simulink model "demo2"  (R2022a)
settings: Solver=ode45  StartTime=0.0  StopTime=inf  RelTol=1e-3  EnableMultiTasking=on
values from neighbouring files (symbols this model uses):
  Cf = 435.418/0.296296    (= 1469.53721954)    [demo2_CM.m]
  controlConstraints = [ ... (first row only)    [demo2_CM.m]
  controlWeight = [1e-7 1e-10 1e-10]    [demo2_CM.m]
  Cr = 756.349/(0.6*pi/180)    (= 72226.0092316)    [demo2_CM.m]
  initial_input = [0 0 0]'    [demo2_CM.m]
  initial_state = [50/3.6 0 0]'    [demo2_CM.m]
  Iz = 2488.892    [demo2_CM.m]
  Kd = 0.0    (= 0)    [demo2_CM.m]
  Ki = 5    [demo2_CM.m]
  Kp = 0.000000005    (= 5e-09)    [demo2_CM.m]
  lf = 1.240    (= 1.24)    [demo2_CM.m]
  lr = 1.510    (= 1.51)    [demo2_CM.m]
  m = 1644.80    (= 1644.8)    [demo2_CM.m]
  Nc = 1    [demo2_CM.m]
  Np = 20    [demo2_CM.m]
  stateConstraints = [ ... (first row only)    [demo2_CM.m]
  stateWeight = [1 1 5]    [demo2_CM.m]
  Ts = 0.01    [demo2_CM.m]
  Vx_ref = 60 / 3.6    (= 16.6666666667)    [demo2_CM.m]
  Vy_ref = 0    [demo2_CM.m]
  w = 0.8    [demo2_CM.m]
  YawRate_ref = -0.006    [demo2_CM.m]
undefined symbols (not defined in the file or in its folder): DiscIntNeverNeededParam, steer
libraries: CarMaker4SL x14, slpidlib x2, simulink x1
(part 2 of 2)

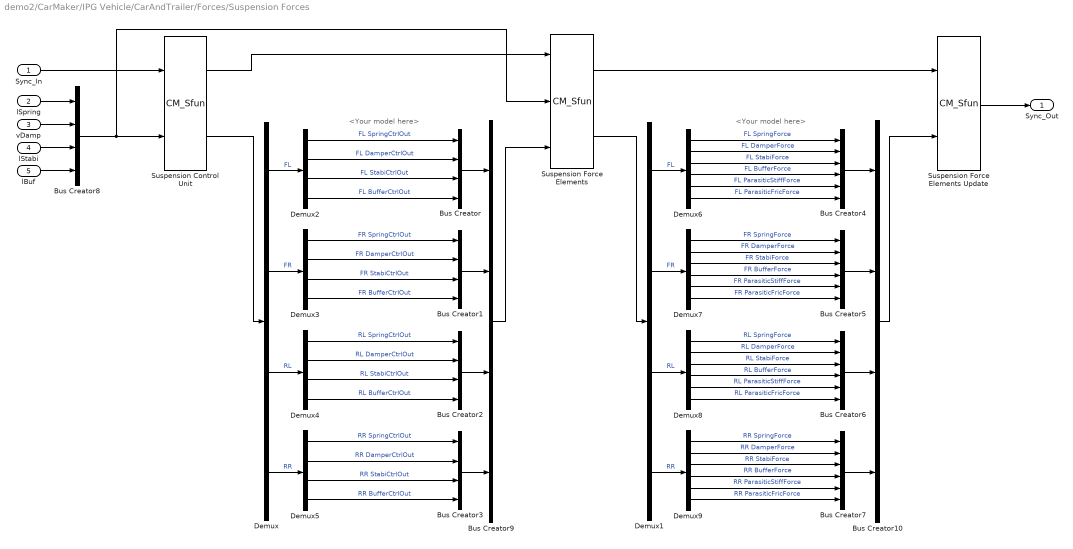
== system demo2/CarMaker/IPG Vehicle/CarAndTrailer/Forces/Suspension Forces ==
  note: <Your model here>
  note: <Your model here>
  Sync_In : Inport
  lSpring : Inport  Port=2
  vDamp : Inport  Port=3
  lStabi : Inport  Port=4
  lBuf : Inport  Port=5
  Bus Creator{,1..3,8..10} (7 alike) : BusCreator  Inputs=4
  Bus Creator{4..7} (4 alike) : BusCreator  Inputs=6
  Demux{,1..5} (6 alike) : Demux
  Demux{6..9} (4 alike) : Demux  Outputs=6
  Suspension Control Unit : S-Function  FunctionName=CM_Sfun  Parameters='ForcesSuspControl'  SFunctionDeploymentMode=off  EnableBusSupport=off
  Suspension Force Elements : S-Function  FunctionName=CM_Sfun  Parameters='ForcesSusp'  SFunctionDeploymentMode=off  EnableBusSupport=off
  Suspension Force Elements Update : S-Function  FunctionName=CM_Sfun  Parameters='ForcesSuspUpd'  SFunctionDeploymentMode=off  EnableBusSupport=off
  Sync_Out : Outport  VectorParamsAs1DForOutWhenUnconnected=off
  wires:
  vDamp/1 -> Bus Creator8/2
  lStabi/1 -> Bus Creator8/3
  lBuf/1 -> Bus Creator8/4
  lSpring/1 -> Bus Creator8/1
  Bus Creator8/1 -> Suspension Control Unit/2, Suspension Force Elements/2
  Sync_In/1 -> Suspension Control Unit/1
  Suspension Control Unit/1 -> Suspension Force Elements/1
  Suspension Force Elements/1 -> Suspension Force Elements Update/1
  Suspension Force Elements Update/1 -> Sync_Out/1
  Bus Creator4/1 -> Bus Creator10/1
  Bus Creator5/1 -> Bus Creator10/2
  Bus Creator6/1 -> Bus Creator10/3
  Bus Creator7/1 -> Bus Creator10/4
  Demux6/1 -> Bus Creator4/1  "FL SpringForce"
  Demux9/1 -> Bus Creator7/1  "RR SpringForce"
  Demux9/2 -> Bus Creator7/2  "RR DamperForce"
  Demux9/3 -> Bus Creator7/3  "RR StabiForce"
  Demux9/4 -> Bus Creator7/4  "RR BufferForce"
  Demux9/5 -> Bus Creator7/5  "RR ParasiticStiffForce"
  Demux9/6 -> Bus Creator7/6  "RR ParasiticFricForce"
  Demux8/1 -> Bus Creator6/1  "RL SpringForce"
  Demux8/2 -> Bus Creator6/2  "RL DamperForce"
  Demux8/4 -> Bus Creator6/4  "RL BufferForce"
  Demux8/5 -> Bus Creator6/5  "RL ParasiticStiffForce"
  Demux8/6 -> Bus Creator6/6  "RL ParasiticFricForce"
  Demux8/3 -> Bus Creator6/3  "RL StabiForce"
  Demux7/1 -> Bus Creator5/1  "FR SpringForce"
  Demux7/2 -> Bus Creator5/2  "FR DamperForce"
  Demux7/3 -> Bus Creator5/3  "FR StabiForce"
  Demux7/4 -> Bus Creator5/4  "FR BufferForce"
  Demux7/5 -> Bus Creator5/5  "FR ParasiticStiffForce"
  Demux7/6 -> Bus Creator5/6  "FR ParasiticFricForce"
  Demux6/2 -> Bus Creator4/2  "FL DamperForce"
  Demux6/3 -> Bus Creator4/3  "FL StabiForce"
  Demux6/4 -> Bus Creator4/4  "FL BufferForce"
  Demux6/5 -> Bus Creator4/5  "FL ParasiticStiffForce"
  Demux6/6 -> Bus Creator4/6  "FL ParasiticFricForce"
  Bus Creator10/1 -> Suspension Force Elements Update/2
  Demux/1 -> Demux2/1  "FL"
  Bus Creator1/1 -> Bus Creator9/2
  Demux/2 -> Demux3/1  "FR"
  Bus Creator2/1 -> Bus Creator9/3
  Demux/3 -> Demux4/1  "RL"
  Bus Creator3/1 -> Bus Creator9/4
  Demux2/1 -> Bus Creator/1  "FL SpringCtrlOut"
  Demux/4 -> Demux5/1  "RR"
  Demux5/1 -> Bus Creator3/1  "RR SpringCtrlOut"
  Demux5/2 -> Bus Creator3/2  "RR DamperCtrlOut"
  Demux5/3 -> Bus Creator3/3  "RR StabiCtrlOut"
  Demux5/4 -> Bus Creator3/4  "RR BufferCtrlOut"
  Demux4/1 -> Bus Creator2/1  "RL SpringCtrlOut"
  Demux4/2 -> Bus Creator2/2  "RL DamperCtrlOut"
  Demux4/4 -> Bus Creator2/4  "RL BufferCtrlOut"
  Demux4/3 -> Bus Creator2/3  "RL StabiCtrlOut"
  Demux3/1 -> Bus Creator1/1  "FR SpringCtrlOut"
  Demux3/2 -> Bus Creator1/2  "FR DamperCtrlOut"
  Demux3/3 -> Bus Creator1/3  "FR StabiCtrlOut"
  Demux3/4 -> Bus Creator1/4  "FR BufferCtrlOut"
  Demux2/2 -> Bus Creator/2  "FL DamperCtrlOut"
  Demux2/3 -> Bus Creator/3  "FL StabiCtrlOut"
  Demux2/4 -> Bus Creator/4  "FL BufferCtrlOut"
  Suspension Control Unit/2 -> Demux/1
  Bus Creator9/1 -> Suspension Force Elements/3
  Bus Creator/1 -> Bus Creator9/1
  Suspension Force Elements/2 -> Demux1/1
  Demux1/1 -> Demux6/1  "FL"
  Demux1/2 -> Demux7/1  "FR"
  Demux1/3 -> Demux8/1  "RL"
  Demux1/4 -> Demux9/1  "RR"

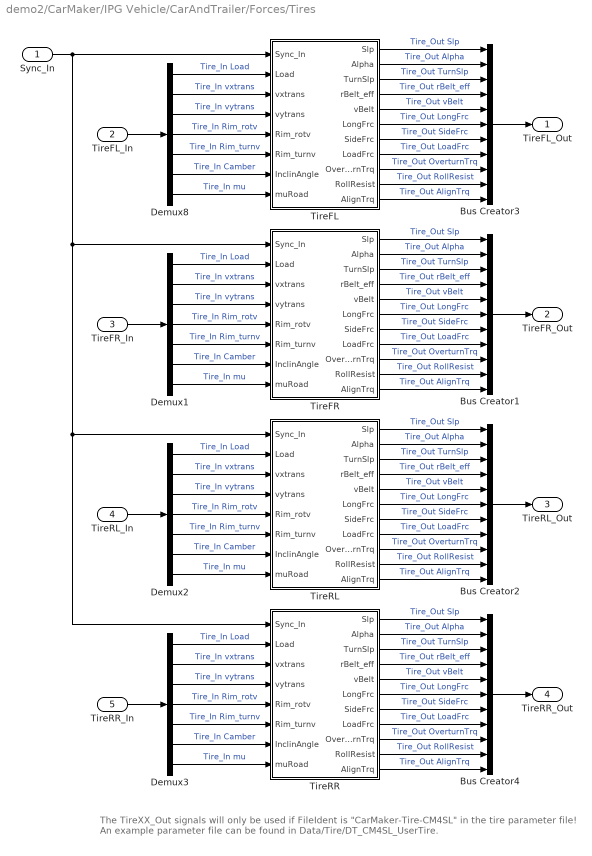
== system demo2/CarMaker/IPG Vehicle/CarAndTrailer/Forces/Tires ==
  note: The TireXX_Out signals will only be used if FileIdent is "CarMaker-Tire-CM4SL" in the tire parameter file!
      | An example parameter file can be found in Data/Tire/DT_CM4SL_UserTire.
  Sync_In : Inport
  TireFL_In : Inport  Port=2
  TireFR_In : Inport  Port=3
  TireRL_In : Inport  Port=4
  TireRR_In : Inport  Port=5
  Bus Creator{1..4} (4 alike) : BusCreator  Inputs=11
  Demux{1..3,8} (4 alike) : Demux  Outputs=7
      settings: DisplayOption=none
  TireFL : Subsystem
  TireFR : Subsystem
  TireRL : Subsystem
  TireRR : Subsystem
  TireFL_Out : Outport  VectorParamsAs1DForOutWhenUnconnected=off
  TireFR_Out : Outport  Port=2  VectorParamsAs1DForOutWhenUnconnected=off
  TireRL_Out : Outport  Port=3  VectorParamsAs1DForOutWhenUnconnected=off
  TireRR_Out : Outport  Port=4  VectorParamsAs1DForOutWhenUnconnected=off
  wires:
  Sync_In/1 -> TireRR/1(Sync_In), TireRL/1(Sync_In), TireFR/1(Sync_In), TireFL/1(Sync_In)
  Bus Creator4/1 -> TireRR_Out/1
  Bus Creator2/1 -> TireRL_Out/1
  Bus Creator1/1 -> TireFR_Out/1
  Demux3/5 -> TireRR/6(Rim_turnv)  "Tire_In Rim_turnv"
  Demux3/4 -> TireRR/5(Rim_rotv)  "Tire_In Rim_rotv"
  Demux3/1 -> TireRR/2(Load)  "Tire_In Load"
  Demux3/7 -> TireRR/8(muRoad)  "Tire_In mu"
  Demux3/6 -> TireRR/7(InclinAngle)  "Tire_In Camber"
  Demux3/2 -> TireRR/3(vxtrans)  "Tire_In vxtrans"
  Demux3/3 -> TireRR/4(vytrans)  "Tire_In vytrans"
  TireRR/11(AlignTrq) -> Bus Creator4/11  "Tire_Out AlignTrq"
  TireRR/10(RollResist) -> Bus Creator4/10  "Tire_Out RollResist"
  TireRR/9(OverturnTrq) -> Bus Creator4/9  "Tire_Out OverturnTrq"
  TireRR/8(LoadFrc) -> Bus Creator4/8  "Tire_Out LoadFrc"
  TireRR/7(SideFrc) -> Bus Creator4/7  "Tire_Out SideFrc"
  TireRR/6(LongFrc) -> Bus Creator4/6  "Tire_Out LongFrc"
  TireRR/5(vBelt) -> Bus Creator4/5  "Tire_Out vBelt"
  TireRR/4(rBelt_eff) -> Bus Creator4/4  "Tire_Out rBelt_eff"
  TireRR/3(TurnSlp) -> Bus Creator4/3  "Tire_Out TurnSlp"
  TireRR/1(Slp) -> Bus Creator4/1  "Tire_Out Slp"
  TireRR/2(Alpha) -> Bus Creator4/2  "Tire_Out Alpha"
  Demux2/5 -> TireRL/6(Rim_turnv)  "Tire_In Rim_turnv"
  Demux2/4 -> TireRL/5(Rim_rotv)  "Tire_In Rim_rotv"
  Demux2/1 -> TireRL/2(Load)  "Tire_In Load"
  Demux2/7 -> TireRL/8(muRoad)  "Tire_In mu"
  Demux2/6 -> TireRL/7(InclinAngle)  "Tire_In Camber"
  Demux2/2 -> TireRL/3(vxtrans)  "Tire_In vxtrans"
  Demux2/3 -> TireRL/4(vytrans)  "Tire_In vytrans"
  TireRL/11(AlignTrq) -> Bus Creator2/11  "Tire_Out AlignTrq"
  TireRL/10(RollResist) -> Bus Creator2/10  "Tire_Out RollResist"
  TireRL/9(OverturnTrq) -> Bus Creator2/9  "Tire_Out OverturnTrq"
  TireRL/8(LoadFrc) -> Bus Creator2/8  "Tire_Out LoadFrc"
  TireRL/7(SideFrc) -> Bus Creator2/7  "Tire_Out SideFrc"
  TireRL/6(LongFrc) -> Bus Creator2/6  "Tire_Out LongFrc"
  TireRL/5(vBelt) -> Bus Creator2/5  "Tire_Out vBelt"
  TireRL/4(rBelt_eff) -> Bus Creator2/4  "Tire_Out rBelt_eff"
  TireRL/3(TurnSlp) -> Bus Creator2/3  "Tire_Out TurnSlp"
  TireRL/1(Slp) -> Bus Creator2/1  "Tire_Out Slp"
  TireRL/2(Alpha) -> Bus Creator2/2  "Tire_Out Alpha"
  Demux1/5 -> TireFR/6(Rim_turnv)  "Tire_In Rim_turnv"
  Demux1/4 -> TireFR/5(Rim_rotv)  "Tire_In Rim_rotv"
  Demux1/1 -> TireFR/2(Load)  "Tire_In Load"
  Demux1/7 -> TireFR/8(muRoad)  "Tire_In mu"
  Demux1/6 -> TireFR/7(InclinAngle)  "Tire_In Camber"
  Demux1/2 -> TireFR/3(vxtrans)  "Tire_In vxtrans"
  Demux1/3 -> TireFR/4(vytrans)  "Tire_In vytrans"
  TireFR/11(AlignTrq) -> Bus Creator1/11  "Tire_Out AlignTrq"
  TireFR/10(RollResist) -> Bus Creator1/10  "Tire_Out RollResist"
  TireFR/9(OverturnTrq) -> Bus Creator1/9  "Tire_Out OverturnTrq"
  TireFR/8(LoadFrc) -> Bus Creator1/8  "Tire_Out LoadFrc"
  TireFR/7(SideFrc) -> Bus Creator1/7  "Tire_Out SideFrc"
  TireFR/6(LongFrc) -> Bus Creator1/6  "Tire_Out LongFrc"
  TireFR/5(vBelt) -> Bus Creator1/5  "Tire_Out vBelt"
  TireFR/4(rBelt_eff) -> Bus Creator1/4  "Tire_Out rBelt_eff"
  TireFR/3(TurnSlp) -> Bus Creator1/3  "Tire_Out TurnSlp"
  TireFR/1(Slp) -> Bus Creator1/1  "Tire_Out Slp"
  TireFR/2(Alpha) -> Bus Creator1/2  "Tire_Out Alpha"
  Demux8/5 -> TireFL/6(Rim_turnv)  "Tire_In Rim_turnv"
  Demux8/4 -> TireFL/5(Rim_rotv)  "Tire_In Rim_rotv"
  TireFL_In/1 -> Demux8/1
  Demux8/1 -> TireFL/2(Load)  "Tire_In Load"
  Demux8/7 -> TireFL/8(muRoad)  "Tire_In mu"
  Demux8/6 -> TireFL/7(InclinAngle)  "Tire_In Camber"
  Demux8/2 -> TireFL/3(vxtrans)  "Tire_In vxtrans"
  Demux8/3 -> TireFL/4(vytrans)  "Tire_In vytrans"
  TireFL/11(AlignTrq) -> Bus Creator3/11  "Tire_Out AlignTrq"
  TireFL/10(RollResist) -> Bus Creator3/10  "Tire_Out RollResist"
  TireFL/9(OverturnTrq) -> Bus Creator3/9  "Tire_Out OverturnTrq"
  TireFL/8(LoadFrc) -> Bus Creator3/8  "Tire_Out LoadFrc"
  TireFL/7(SideFrc) -> Bus Creator3/7  "Tire_Out SideFrc"
  TireFL/6(LongFrc) -> Bus Creator3/6  "Tire_Out LongFrc"
  TireFL/5(vBelt) -> Bus Creator3/5  "Tire_Out vBelt"
  TireFL/4(rBelt_eff) -> Bus Creator3/4  "Tire_Out rBelt_eff"
  TireFL/3(TurnSlp) -> Bus Creator3/3  "Tire_Out TurnSlp"
  TireFL/1(Slp) -> Bus Creator3/1  "Tire_Out Slp"
  TireFL/2(Alpha) -> Bus Creator3/2  "Tire_Out Alpha"
  Bus Creator3/1 -> TireFL_Out/1
  TireFR_In/1 -> Demux1/1
  TireRL_In/1 -> Demux2/1
  TireRR_In/1 -> Demux3/1

== system demo2/CarMaker/IPG Vehicle/CarAndTrailer/Forces/Vehicle Forces ==
  Sync_In : Inport
  Bus Creator1 : BusCreator  Inputs=12
  Bus Creator8 : BusCreator  Inputs=16
  BusCreator1 : BusCreator  Inputs=4
  BusCreator2 : BusCreator  Inputs=9
  Demux : Demux  Outputs=16
      settings: DisplayOption=none
  Demux1 : Demux  Outputs=12
      settings: DisplayOption=none
  Demux2 : Demux  Outputs=13
      settings: DisplayOption=none
  Forces : S-Function  FunctionName=CM_Sfun  Parameters='Forces'  SFunctionDeploymentMode=off  EnableBusSupport=off
  Terminator : Terminator
  Sync_Out : Outport  VectorParamsAs1DForOutWhenUnconnected=off
  Car.Virtual : Outport  Port=2  VectorParamsAs1DForOutWhenUnconnected=off
  Car.Aero : Outport  Port=3  VectorParamsAs1DForOutWhenUnconnected=off
  Car.Load : Outport  Port=4  VectorParamsAs1DForOutWhenUnconnected=off
  wires:
  BusCreator1/1 -> Terminator/1  "Aero IF (in)"
  Demux2/13 -> BusCreator2/9  "car Aero Trq_1 z"
  Demux2/12 -> BusCreator2/8  "car Aero Trq_1 y"
  Demux2/11 -> BusCreator2/7  "car Aero Trq_1 x"
  Demux2/10 -> BusCreator2/6  "car Aero Frc_1 z"
  Demux2/9 -> BusCreator2/5  "car Aero Frc_1 y"
  Demux2/8 -> BusCreator2/4  "car Aero Frc_1 x"
  Demux2/7 -> BusCreator2/3  "car Aero PoA_1 z"
  Demux2/6 -> BusCreator2/2  "car Aero PoA_1 y"
  Demux2/5 -> BusCreator2/1  "car Aero PoA_1 x"
  Demux2/4 -> BusCreator1/4  "car Aero tau_1"
  Demux2/3 -> BusCreator1/3  "car Aero ApproachVel_1 z"
  Demux2/2 -> BusCreator1/2  "car Aero ApproachVel_1 y"
  Demux2/1 -> BusCreator1/1  "car Aero ApproachVel_1 x"
  Demux/16 -> Bus Creator8/16  "Car Load_3 tz"
  Demux/15 -> Bus Creator8/15  "Car Load_3 ty"
  Demux/14 -> Bus Creator8/14  "Car Load_3 tx"
  Demux/13 -> Bus Creator8/13  "Car Load_3 mass"
  Demux1/12 -> Bus Creator1/12  "Car Virtual Trq_0 z"
  Demux1/11 -> Bus Creator1/11  "Car Virtual Trq_0 y"
  Demux1/10 -> Bus Creator1/10  "Car Virtual Trq_0 x"
  Demux1/9 -> Bus Creator1/9  "Car Virtual Trq_1 z"
  Demux1/8 -> Bus Creator1/8  "Car Virtual Trq_1 y"
  Demux1/7 -> Bus Creator1/7  "Car Virtual Trq_1 x"
  Demux1/6 -> Bus Creator1/6  "Car Virtual Frc_0 z"
  Demux1/5 -> Bus Creator1/5  "Car Virtual Frc_0 y"
  Demux1/4 -> Bus Creator1/4  "Car Virtual Frc_0 x"
  Sync_In/1 -> Forces/1
  Forces/1 -> Sync_Out/1
  BusCreator2/1 -> Car.Aero/1
  Demux1/1 -> Bus Creator1/1  "Car Virtual Frc_1 x"
  Demux1/2 -> Bus Creator1/2  "Car Virtual Frc_1 y"
  Demux1/3 -> Bus Creator1/3  "Car Virtual Frc_1 z"
  Forces/3 -> Demux2/1
  Forces/2 -> Demux1/1
  Bus Creator1/1 -> Car.Virtual/1
  Bus Creator8/1 -> Car.Load/1
  Demux/1 -> Bus Creator8/1  "Car Load_0 mass"
  Demux/2 -> Bus Creator8/2  "Car Load_0 tx"
  Demux/3 -> Bus Creator8/3  "Car Load_0 ty"
  Demux/4 -> Bus Creator8/4  "Car Load_0 tz"
  Demux/5 -> Bus Creator8/5  "Car Load_1 mass"
  Demux/6 -> Bus Creator8/6  "Car Load_1 tx"
  Demux/7 -> Bus Creator8/7  "Car Load_1 ty"
  Demux/8 -> Bus Creator8/8  "Car Load_1 tz"
  Demux/9 -> Bus Creator8/9  "Car Load_2 mass"
  Demux/10 -> Bus Creator8/10  "Car Load_2 tx"
  Demux/11 -> Bus Creator8/11  "Car Load_2 ty"
  Demux/12 -> Bus Creator8/12  "Car Load_2 tz"
  Forces/4 -> Demux/1

== system demo2/CarMaker/IPG Vehicle/CarAndTrailer/Trailer/CreateBus Car.Hitch.FrcTrq ==
  In1 : Inport
  Bus Creator7 : BusCreator  Inputs=6
  Demux7 : Demux  Outputs=6
      settings: DisplayOption=none
  Out1 : Outport  VectorParamsAs1DForOutWhenUnconnected=off
  wires:
  In1/1 -> Demux7/1
  Bus Creator7/1 -> Out1/1
  Demux7/6 -> Bus Creator7/6  "Car Hitch Trq2Car z"
  Demux7/5 -> Bus Creator7/5  "Car Hitch Trq2Car y"
  Demux7/4 -> Bus Creator7/4  "Car Hitch Trq2Car x"
  Demux7/3 -> Bus Creator7/3  "Car Hitch Frc2Car z"
  Demux7/2 -> Bus Creator7/2  "Car Hitch Frc2Car y"
  Demux7/1 -> Bus Creator7/1  "Car Hitch Frc2Car x"

== system demo2/CarMaker/IPG Vehicle/CarAndTrailer/Trailer/CreateBus Vhcl.Motion ==
  In1 : Inport
  BusCreator : BusCreator  Inputs=15
  Demux : Demux  Outputs=15
      settings: DisplayOption=none
  Out1 : Outport  VectorParamsAs1DForOutWhenUnconnected=off
  wires:
  Demux/15 -> BusCreator/15  "Vhcl YawAcc"
  Demux/14 -> BusCreator/14  "Vhcl YawVel"
  Demux/13 -> BusCreator/13  "Vhcl Yaw"
  Demux/12 -> BusCreator/12  "Vhcl PitchAcc"
  Demux/11 -> BusCreator/11  "Vhcl PitchVel"
  Demux/10 -> BusCreator/10  "Vhcl Pitch"
  Demux/9 -> BusCreator/9  "Vhcl RollAcc"
  Demux/8 -> BusCreator/8  "Vhcl RollVel"
  Demux/7 -> BusCreator/7  "Vhcl Roll"
  Demux/6 -> BusCreator/6  "Vhcl Hitch_Pos z"
  Demux/5 -> BusCreator/5  "Vhcl Hitch_Pos y"
  Demux/4 -> BusCreator/4  "Vhcl Hitch_Pos x"
  Demux/3 -> BusCreator/3  "Vhcl sRoad"
  Demux/2 -> BusCreator/2  "Vhcl Distance"
  Demux/1 -> BusCreator/1  "Vhcl v"
  In1/1 -> Demux/1
  BusCreator/1 -> Out1/1

== system demo2/CarMaker/IPG Vehicle/CarAndTrailer/Trailer/CreateBus Vhcl.PoI ==
  In1 : Inport
  Bus Creator3 : BusCreator  Inputs=18
  Demux3 : Demux  Outputs=18
      settings: DisplayOption=none
  Out1 : Outport  VectorParamsAs1DForOutWhenUnconnected=off
  wires:
  Demux3/18 -> Bus Creator3/18  "Vhcl PoI_GCS Elev"
  Demux3/17 -> Bus Creator3/17  "Vhcl PoI_GCS Lat"
  Demux3/16 -> Bus Creator3/16  "Vhcl PoI_GCS Long"
  Demux3/15 -> Bus Creator3/15  "Vhcl PoI_Acc_1 z"
  Demux3/14 -> Bus Creator3/14  "Vhcl PoI_Acc_1 y"
  Demux3/13 -> Bus Creator3/13  "Vhcl PoI_Acc_1 x"
  Demux3/12 -> Bus Creator3/12  "Vhcl PoI_Vel_1 z"
  Demux3/11 -> Bus Creator3/11  "Vhcl PoI_Vel_1 y"
  Demux3/10 -> Bus Creator3/10  "Vhcl PoI_Vel_1 x"
  Demux3/9 -> Bus Creator3/9  "Vhcl PoI_Acc z"
  Demux3/8 -> Bus Creator3/8  "Vhcl PoI_Acc y"
  Demux3/7 -> Bus Creator3/7  "Vhcl PoI_Acc x"
  Demux3/6 -> Bus Creator3/6  "Vhcl PoI_Vel z"
  Demux3/5 -> Bus Creator3/5  "Vhcl PoI_Vel y"
  Demux3/4 -> Bus Creator3/4  "Vhcl PoI_Vel x"
  Demux3/3 -> Bus Creator3/3  "Vhcl PoI_Pos z"
  Demux3/2 -> Bus Creator3/2  "Vhcl PoI_Pos y"
  In1/1 -> Demux3/1
  Bus Creator3/1 -> Out1/1
  Demux3/1 -> Bus Creator3/1  "Vhcl PoI_Pos x"

== system demo2/CarMaker/IPG Vehicle/CarAndTrailer/Trailer/CreateBus Vhcl.Steering ==
  In1 : Inport
  Bus Creator3 : BusCreator  Inputs=4
  Demux : Demux
      settings: DisplayOption=none
  Out1 : Outport  VectorParamsAs1DForOutWhenUnconnected=off
  wires:
  Bus Creator3/1 -> Out1/1
  Demux/1 -> Bus Creator3/1  "Vhcl Steering Ang"
  Demux/3 -> Bus Creator3/3  "Vhcl Steering AngAcc"
  Demux/2 -> Bus Creator3/2  "Vhcl Steering AngVel"
  Demux/4 -> Bus Creator3/4  "Vhcl Steering Trq"
  In1/1 -> Demux/1

== system demo2/CarMaker/IPG Vehicle/CarAndTrailer/Trailer/CreateBus Vhcl.Wheel.FL ==
  In1 : Inport
  Bus Creator3 : BusCreator  Inputs=14
  Demux3 : Demux  Outputs=14
      settings: DisplayOption=none
  Out1 : Outport  VectorParamsAs1DForOutWhenUnconnected=off
  wires:
  Demux3/14 -> Bus Creator3/14  "Vhcl Wheel FL Trq_WhlBearing"
  Demux3/13 -> Bus Creator3/13  "Vhcl Wheel FL Trq_T2W"
  Demux3/12 -> Bus Creator3/12  "Vhcl Wheel FL SideSlip"
  Demux3/11 -> Bus Creator3/11  "Vhcl Wheel FL LongSlip"
  Demux3/10 -> Bus Creator3/10  "Vhcl Wheel FL vBelt"
  Demux3/9 -> Bus Creator3/9  "Vhcl Wheel FL Fz"
  Demux3/8 -> Bus Creator3/8  "Vhcl Wheel FL Fy"
  Demux3/7 -> Bus Creator3/7  "Vhcl Wheel FL F"
  Demux3/6 -> Bus Creator3/6  "Vhcl Wheel FL r_zxy z"
  Demux3/5 -> Bus Creator3/5  "Vhcl Wheel FL r_zxy y"
  Demux3/4 -> Bus Creator3/4  "Vhcl Wheel FL r_zxy x"
  Demux3/3 -> Bus Creator3/3  "Vhcl Wheel FL t z"
  Demux3/2 -> Bus Creator3/2  "Vhcl Wheel FL t y"
  In1/1 -> Demux3/1
  Bus Creator3/1 -> Out1/1
  Demux3/1 -> Bus Creator3/1  "Vhcl Wheel FL t x"

== system demo2/CarMaker/IPG Vehicle/CarAndTrailer/Trailer/CreateBus Vhcl.Wheel.FR ==
  In1 : Inport
  Bus Creator3 : BusCreator  Inputs=14
  Demux3 : Demux  Outputs=14
      settings: DisplayOption=none
  Out1 : Outport  VectorParamsAs1DForOutWhenUnconnected=off
  wires:
  Demux3/14 -> Bus Creator3/14  "Vhcl Wheel FR Trq_WhlBearing"
  Demux3/13 -> Bus Creator3/13  "Vhcl Wheel FR Trq_T2W"
  Demux3/12 -> Bus Creator3/12  "Vhcl Wheel FR SideSlip"
  Demux3/11 -> Bus Creator3/11  "Vhcl Wheel FR LongSlip"
  Demux3/10 -> Bus Creator3/10  "Vhcl Wheel FR vBelt"
  Demux3/9 -> Bus Creator3/9  "Vhcl Wheel FR Fz"
  Demux3/8 -> Bus Creator3/8  "Vhcl Wheel FR Fy"
  Demux3/7 -> Bus Creator3/7  "Vhcl Wheel FR Fx"
  Demux3/6 -> Bus Creator3/6  "Vhcl Wheel FR r_zxy z"
  Demux3/5 -> Bus Creator3/5  "Vhcl Wheel FR r_zxy y"
  Demux3/4 -> Bus Creator3/4  "Vhcl Wheel FR r_zxy x"
  Demux3/3 -> Bus Creator3/3  "Vhcl Wheel FR t z"
  Demux3/2 -> Bus Creator3/2  "Vhcl Wheel FR t y"
  In1/1 -> Demux3/1
  Bus Creator3/1 -> Out1/1
  Demux3/1 -> Bus Creator3/1  "Vhcl Wheel FR t x"

== system demo2/CarMaker/IPG Vehicle/CarAndTrailer/Trailer/CreateBus Vhcl.Wheel.RL ==
  In1 : Inport
  Bus Creator3 : BusCreator  Inputs=14
  Demux3 : Demux  Outputs=14
      settings: DisplayOption=none
  Out1 : Outport  VectorParamsAs1DForOutWhenUnconnected=off
  wires:
  Demux3/14 -> Bus Creator3/14  "Vhcl Wheel RL Trq_WhlBearing"
  Demux3/13 -> Bus Creator3/13  "Vhcl Wheel RL Trq_T2W"
  Demux3/12 -> Bus Creator3/12  "Vhcl Wheel RL SideSlip"
  Demux3/11 -> Bus Creator3/11  "Vhcl Wheel RL LongSlip"
  Demux3/10 -> Bus Creator3/10  "Vhcl Wheel RL vBelt"
  Demux3/9 -> Bus Creator3/9  "Vhcl Wheel RL Fz"
  Demux3/8 -> Bus Creator3/8  "Vhcl Wheel RL Fy"
  Demux3/7 -> Bus Creator3/7  "Vhcl Wheel RL Fx"
  Demux3/6 -> Bus Creator3/6  "Vhcl Wheel RL r_zxy z"
  Demux3/5 -> Bus Creator3/5  "Vhcl Wheel RL r_zxy y"
  Demux3/4 -> Bus Creator3/4  "Vhcl Wheel RL r_zxy x"
  Demux3/3 -> Bus Creator3/3  "Vhcl Wheel RL t z"
  Demux3/2 -> Bus Creator3/2  "Vhcl Wheel RL t y"
  In1/1 -> Demux3/1
  Bus Creator3/1 -> Out1/1
  Demux3/1 -> Bus Creator3/1  "Vhcl Wheel RL t x"

== system demo2/CarMaker/IPG Vehicle/CarAndTrailer/Trailer/CreateBus Vhcl.Wheel.RR ==
  In1 : Inport
  Bus Creator3 : BusCreator  Inputs=14
  Demux3 : Demux  Outputs=14
      settings: DisplayOption=none
  Out1 : Outport  VectorParamsAs1DForOutWhenUnconnected=off
  wires:
  Demux3/14 -> Bus Creator3/14  "Vhcl Wheel RR Trq_WhlBearing"
  Demux3/13 -> Bus Creator3/13  "Vhcl Wheel RR Trq_T2W"
  Demux3/12 -> Bus Creator3/12  "Vhcl Wheel RR SideSlip"
  Demux3/11 -> Bus Creator3/11  "Vhcl Wheel RR LongSlip"
  Demux3/10 -> Bus Creator3/10  "Vhcl Wheel RR vBelt"
  Demux3/9 -> Bus Creator3/9  "Vhcl Wheel RR Fz"
  Demux3/8 -> Bus Creator3/8  "Vhcl Wheel RR Fy"
  Demux3/7 -> Bus Creator3/7  "Vhcl Wheel RR Fx"
  Demux3/6 -> Bus Creator3/6  "Vhcl Wheel RR r_zxy z"
  Demux3/5 -> Bus Creator3/5  "Vhcl Wheel RR r_zxy y"
  Demux3/4 -> Bus Creator3/4  "Vhcl Wheel RR r_zxy x"
  Demux3/3 -> Bus Creator3/3  "Vhcl Wheel RR t z"
  Demux3/2 -> Bus Creator3/2  "Vhcl Wheel RR t y"
  In1/1 -> Demux3/1
  Bus Creator3/1 -> Out1/1
  Demux3/1 -> Bus Creator3/1  "Vhcl Wheel RR t x"

== system demo2/CarMaker/VehicleControl/CreateBus VhclCtrl/MPC Controller/Adaptive MPC ==
  state : Inport
  ref : Inport  Port=2
  Delay One Step : Delay  DelayLength=1
  Delay One Step2 : Delay  DelayLength=1
  Discrete-Time Integrator1 : DiscreteIntegrator  IntegratorMethod=Integration: Backward Euler  SampleTime=Ts  ICPrevOutput=DiscIntNeverNeededParam  ICPrevScaledInput=DiscIntNeverNeededParam
  IC : InitialCondition  Value=initial_input
  IC1 : InitialCondition  Value=initial_state
  Linearization : Subsystem
  MPC Main Function : MATLAB Function  TreatAsAtomicUnit=on  SystemSampleTime=Ts
  Plus : Sum  Inputs=+-
  Reshape1 : Reshape  OutputDimensionality=Column vector (2-D)
  Reshape3 : Reshape  OutputDimensionality=Column vector (2-D)
  Selector : Selector  InputPortWidth=3  IndexOptions=Index vector (dialog)  Indices=[1:3]  OutputSizes=1
  "delta input " : Outport
  input : Outport  Port=2
  wires:
  Delay One Step/1 -> Plus/2
  Plus/1 -> MPC Main Function/5(delState)
  Selector/1 -> "delta input "/1, Discrete-Time Integrator1/1
  Linearization/2(B) -> MPC Main Function/2(B)
  Linearization/1(A) -> MPC Main Function/1(A)
  ref/1 -> MPC Main Function/7(ref)
  Linearization/3(C) -> MPC Main Function/3(C)
  Reshape1/1 -> IC1/1  "X"
  Reshape3/1 -> input/1, Delay One Step2/1  "X"
  Delay One Step2/1 -> IC/1
  Discrete-Time Integrator1/1 -> Reshape3/1
  IC/1 -> MPC Main Function/6(preInput), Linearization/2(previous input)
  IC1/1 -> MPC Main Function/4(state), Plus/1, Delay One Step/1, Linearization/1(operating state)
  state/1 -> Reshape1/1
  MPC Main Function/1(U) -> Selector/1

== system demo2/CarMaker/VehicleControl/CreateBus VhclCtrl/MPC Controller/PID Controller ==
  input : Inport
  Demux : Demux  Outputs=3
  PID Controller1 : slpidlib/PID Controller  Controller=PID  Form=Parallel  TimeDomain=Continuous-time  UseExternalTs=off  SampleTime=Ts  IntegratorMethod=Forward Euler  FilterMethod=Forward Euler  ControllerParametersSource=internal  P=Kp  I=Ki  UseKiTs=off  D=Kd  N=100  UseFilter=on  TunerSelectOption=Transfer Function Based (PID Tuner App)  InitialConditionSource=internal  InitialConditionForIntegrator=0  InitialConditionForFilter=0  DifferentiatorICPrevScaledInput=0  ExternalReset=none  TrackingMode=off  Kt=1  LimitOutput=off  SatLimitsSource=internal  UpperSaturationLimit=inf  LowerSaturationLimit=-inf  LinearizeAsGain=on  AntiWindupMode=none  Kb=1  POutMin=[]  POutMax=[]  IOutMin=[]  IOutMax=[]  DOutMin=[]  DOutMax=[]  NOutMin=[]  NOutMax=[]  SumOutMin=[]  SumOutMax=[]  SaturationOutMin=[]  SaturationOutMax=[]  PParamMin=[]  PParamMax=[]  IParamMin=[]  IParamMax=[]  DParamMin=[]  DParamMax=[]  NParamMin=[]  NParamMax=[]  KbParamMin=[]  KbParamMax=[]  KtParamMin=[]  KtParamMax=[]  KbOutMin=[]  KbOutMax=[]  KtOutMin=[]  KtOutMax=[]  IntegratorOutMin=[]  IntegratorOutMax=[]  FilterOutMin=[]  FilterOutMax=[]  SumI1OutMin=[]  SumI1OutMax=[]  SumI2OutMin=[]  SumI2OutMax=[]  SumI3OutMin=[]  SumI3OutMax=[]  SumI4OutMin=[]  SumI4OutMax=[]  SumDOutMin=[]  SumDOutMax=[]  DifferentiatorOutMin=[]  DifferentiatorOutMax=[]  FilterDiffOutCoefMin=[]  FilterDiffOutCoefMax=[]  ReciprocalOutMin=[]  ReciprocalOutMax=[]  SumDenOutMin=[]  SumDenOutMax=[]  SumNumOutMin=[]  SumNumOutMax=[]  DivideOutMin=[]  DivideOutMax=[]  UdiffTsProdOutMin=[]  UdiffTsProdOutMax=[]  NTsProdOutMin=[]  NTsProdOutMax=[]  UintegralTsProdOutMin=[]  UintegralTsProdOutMax=[]  UngainTsProdOutMin=[]  UngainTsProdOutMax=[]  ClampingZeroOutDataTypeStr=Inherit: Inherit via back propagation  ClampingZeroOutMin=[]  ClampingZeroOutMax=[]  FilterDenConstantOutDataTypeStr=Inherit: Inherit via back propagation  FilterDenConstantOutMin=[]  FilterDenConstantOutMax=[]  PCopyOutDataTypeStr=Inherit: Inherit via back propagation  PCopyOutMin=[]  PCopyOutMax=[]  NCopyOutDataTypeStr=Inherit: Inherit via back propagation  NCopyOutMin=[]  NCopyOutMax=[]  IntegratorContinuousStateAttributes=''  IntegratorStateMustResolveToSignalObject=off  IntegratorRTWStateStorageClass=Auto  FilterContinuousStateAttributes=''  FilterStateMustResolveToSignalObject=off  FilterRTWStateStorageClass=Auto  ParallelPVariant=InternalParameters  IdealPVariant=Disabled  IVariant=InternalParameters  DVariant=InternalParameters  IntegratorVariant=Continuous  SatVariant=Disabled  AWVariant=Passthrough  PCopyVariant=Disabled  TRVariant=Disabled  FdbkBlocksVariant=Forward  IdealPFdbkVariant=Disabled  SatFdbkVariant=Disabled  DerivativeFilterVariant=ContFilter  NVariant=InternalParameters  NCopyVariant=Disabled  FilterICVariant=InternalICsFilter  IntegratorICVariant=InternalICs  ExternalResetVariant=Disabled  TRSumVariant=Passthrough  SumFdbkVariant=Disabled  SumVariant=Sum_PID  TsampFilterVariant=InternalTs  TsampNgainVariant=Passthrough  TsampIntegralVariant=Passthrough  ExternalSaturationOutDataTypeStr=Inherit: Same as second input  aMode=0
  PID Controller2 : slpidlib/PID Controller  Controller=PID  Form=Parallel  TimeDomain=Continuous-time  UseExternalTs=off  SampleTime=Ts  IntegratorMethod=Forward Euler  FilterMethod=Forward Euler  ControllerParametersSource=internal  P=Kp  I=Ki  UseKiTs=off  D=Kd  N=100  UseFilter=on  TunerSelectOption=Transfer Function Based (PID Tuner App)  InitialConditionSource=internal  InitialConditionForIntegrator=0  InitialConditionForFilter=0  DifferentiatorICPrevScaledInput=0  ExternalReset=none  TrackingMode=off  Kt=1  LimitOutput=off  SatLimitsSource=internal  UpperSaturationLimit=inf  LowerSaturationLimit=-inf  LinearizeAsGain=on  AntiWindupMode=none  Kb=1  POutMin=[]  POutMax=[]  IOutMin=[]  IOutMax=[]  DOutMin=[]  DOutMax=[]  NOutMin=[]  NOutMax=[]  SumOutMin=[]  SumOutMax=[]  SaturationOutMin=[]  SaturationOutMax=[]  PParamMin=[]  PParamMax=[]  IParamMin=[]  IParamMax=[]  DParamMin=[]  DParamMax=[]  NParamMin=[]  NParamMax=[]  KbParamMin=[]  KbParamMax=[]  KtParamMin=[]  KtParamMax=[]  KbOutMin=[]  KbOutMax=[]  KtOutMin=[]  KtOutMax=[]  IntegratorOutMin=[]  IntegratorOutMax=[]  FilterOutMin=[]  FilterOutMax=[]  SumI1OutMin=[]  SumI1OutMax=[]  SumI2OutMin=[]  SumI2OutMax=[]  SumI3OutMin=[]  SumI3OutMax=[]  SumI4OutMin=[]  SumI4OutMax=[]  SumDOutMin=[]  SumDOutMax=[]  DifferentiatorOutMin=[]  DifferentiatorOutMax=[]  FilterDiffOutCoefMin=[]  FilterDiffOutCoefMax=[]  ReciprocalOutMin=[]  ReciprocalOutMax=[]  SumDenOutMin=[]  SumDenOutMax=[]  SumNumOutMin=[]  SumNumOutMax=[]  DivideOutMin=[]  DivideOutMax=[]  UdiffTsProdOutMin=[]  UdiffTsProdOutMax=[]  NTsProdOutMin=[]  NTsProdOutMax=[]  UintegralTsProdOutMin=[]  UintegralTsProdOutMax=[]  UngainTsProdOutMin=[]  UngainTsProdOutMax=[]  ClampingZeroOutDataTypeStr=Inherit: Inherit via back propagation  ClampingZeroOutMin=[]  ClampingZeroOutMax=[]  FilterDenConstantOutDataTypeStr=Inherit: Inherit via back propagation  FilterDenConstantOutMin=[]  FilterDenConstantOutMax=[]  PCopyOutDataTypeStr=Inherit: Inherit via back propagation  PCopyOutMin=[]  PCopyOutMax=[]  NCopyOutDataTypeStr=Inherit: Inherit via back propagation  NCopyOutMin=[]  NCopyOutMax=[]  IntegratorContinuousStateAttributes=''  IntegratorStateMustResolveToSignalObject=off  IntegratorRTWStateStorageClass=Auto  FilterContinuousStateAttributes=''  FilterStateMustResolveToSignalObject=off  FilterRTWStateStorageClass=Auto  ParallelPVariant=InternalParameters  IdealPVariant=Disabled  IVariant=InternalParameters  DVariant=InternalParameters  IntegratorVariant=Continuous  SatVariant=Disabled  AWVariant=Passthrough  PCopyVariant=Disabled  TRVariant=Disabled  FdbkBlocksVariant=Forward  IdealPFdbkVariant=Disabled  SatFdbkVariant=Disabled  DerivativeFilterVariant=ContFilter  NVariant=InternalParameters  NCopyVariant=Disabled  FilterICVariant=InternalICsFilter  IntegratorICVariant=InternalICs  ExternalResetVariant=Disabled  TRSumVariant=Passthrough  SumFdbkVariant=Disabled  SumVariant=Sum_PID  TsampFilterVariant=InternalTs  TsampNgainVariant=Passthrough  TsampIntegralVariant=Passthrough  ExternalSaturationOutDataTypeStr=Inherit: Same as second input  aMode=0
  Read CM Dict8 : CarMaker4SL/Read CM Dict  xname=Vhcl.RL.Fx  xsync=off  xstime=Continuous
  Read CM Dict9 : CarMaker4SL/Read CM Dict  xname=Vhcl.RR.Fx  xsync=off  xstime=Continuous
  Sum1 : Sum  Inputs=|+-
  Sum2 : Sum  Inputs=|+-
  Steering Wheel : Outport
  RL_Torque : Outport  Port=2
  RR_Torque : Outport  Port=3
  wires:
  Sum1/1 -> PID Controller1/1
  Demux/3 -> Sum1/1
  Sum2/1 -> PID Controller2/1
  Demux/2 -> Sum2/1
  input/1 -> Demux/1
  PID Controller2/1 -> RL_Torque/1
  PID Controller1/1 -> RR_Torque/1
  Demux/1 -> Steering Wheel/1
  Read CM Dict8/1 -> Sum2/2
  Read CM Dict9/1 -> Sum1/2

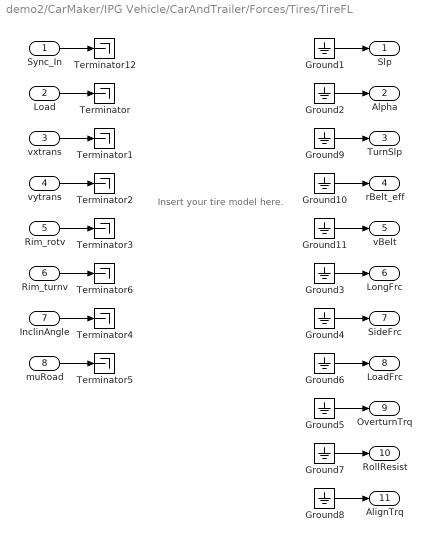
== system demo2/CarMaker/IPG Vehicle/CarAndTrailer/Forces/Tires/TireFL ==
  note: Insert your tire model here.
  Sync_In : Inport
  Load : Inport  Port=2
  vxtrans : Inport  Port=3
  vytrans : Inport  Port=4
  Rim_rotv : Inport  Port=5
  Rim_turnv : Inport  Port=6
  InclinAngle : Inport  Port=7
  muRoad : Inport  Port=8
  Ground{1..11} (11 alike) : Ground
  Terminator{,1..6,12} (8 alike) : Terminator
  Slp : Outport  VectorParamsAs1DForOutWhenUnconnected=off
  Alpha : Outport  Port=2  VectorParamsAs1DForOutWhenUnconnected=off
  TurnSlp : Outport  Port=3  VectorParamsAs1DForOutWhenUnconnected=off
  rBelt_eff : Outport  Port=4  VectorParamsAs1DForOutWhenUnconnected=off
  vBelt : Outport  Port=5  VectorParamsAs1DForOutWhenUnconnected=off
  LongFrc : Outport  Port=6  VectorParamsAs1DForOutWhenUnconnected=off
  SideFrc : Outport  Port=7  VectorParamsAs1DForOutWhenUnconnected=off
  LoadFrc : Outport  Port=8  VectorParamsAs1DForOutWhenUnconnected=off
  OverturnTrq : Outport  Port=9  VectorParamsAs1DForOutWhenUnconnected=off
  RollResist : Outport  Port=10  VectorParamsAs1DForOutWhenUnconnected=off
  AlignTrq : Outport  Port=11  VectorParamsAs1DForOutWhenUnconnected=off
  wires:
  Ground11/1 -> vBelt/1
  Ground10/1 -> rBelt_eff/1
  Ground9/1 -> TurnSlp/1
  Rim_turnv/1 -> Terminator6/1
  Sync_In/1 -> Terminator12/1
  Ground2/1 -> Alpha/1
  Ground3/1 -> LongFrc/1
  Ground4/1 -> SideFrc/1
  Ground5/1 -> OverturnTrq/1
  vxtrans/1 -> Terminator1/1
  vytrans/1 -> Terminator2/1
  Rim_rotv/1 -> Terminator3/1
  InclinAngle/1 -> Terminator4/1
  muRoad/1 -> Terminator5/1
  Load/1 -> Terminator/1
  Ground1/1 -> Slp/1
  Ground6/1 -> LoadFrc/1
  Ground7/1 -> RollResist/1
  Ground8/1 -> AlignTrq/1

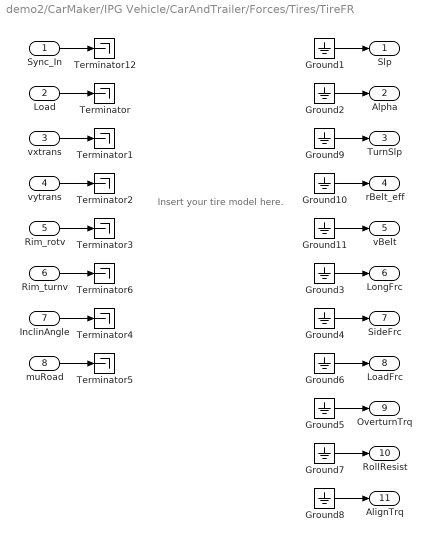
== system demo2/CarMaker/IPG Vehicle/CarAndTrailer/Forces/Tires/TireFR ==
  note: Insert your tire model here.
  Sync_In : Inport
  Load : Inport  Port=2
  vxtrans : Inport  Port=3
  vytrans : Inport  Port=4
  Rim_rotv : Inport  Port=5
  Rim_turnv : Inport  Port=6
  InclinAngle : Inport  Port=7
  muRoad : Inport  Port=8
  Ground{1..11} (11 alike) : Ground
  Terminator{,1..6,12} (8 alike) : Terminator
  Slp : Outport  VectorParamsAs1DForOutWhenUnconnected=off
  Alpha : Outport  Port=2  VectorParamsAs1DForOutWhenUnconnected=off
  TurnSlp : Outport  Port=3  VectorParamsAs1DForOutWhenUnconnected=off
  rBelt_eff : Outport  Port=4  VectorParamsAs1DForOutWhenUnconnected=off
  vBelt : Outport  Port=5  VectorParamsAs1DForOutWhenUnconnected=off
  LongFrc : Outport  Port=6  VectorParamsAs1DForOutWhenUnconnected=off
  SideFrc : Outport  Port=7  VectorParamsAs1DForOutWhenUnconnected=off
  LoadFrc : Outport  Port=8  VectorParamsAs1DForOutWhenUnconnected=off
  OverturnTrq : Outport  Port=9  VectorParamsAs1DForOutWhenUnconnected=off
  RollResist : Outport  Port=10  VectorParamsAs1DForOutWhenUnconnected=off
  AlignTrq : Outport  Port=11  VectorParamsAs1DForOutWhenUnconnected=off
  wires:
  Ground11/1 -> vBelt/1
  Ground10/1 -> rBelt_eff/1
  Ground9/1 -> TurnSlp/1
  Rim_turnv/1 -> Terminator6/1
  Sync_In/1 -> Terminator12/1
  Ground2/1 -> Alpha/1
  Ground3/1 -> LongFrc/1
  Ground4/1 -> SideFrc/1
  Ground5/1 -> OverturnTrq/1
  vxtrans/1 -> Terminator1/1
  vytrans/1 -> Terminator2/1
  Rim_rotv/1 -> Terminator3/1
  InclinAngle/1 -> Terminator4/1
  muRoad/1 -> Terminator5/1
  Load/1 -> Terminator/1
  Ground1/1 -> Slp/1
  Ground6/1 -> LoadFrc/1
  Ground7/1 -> RollResist/1
  Ground8/1 -> AlignTrq/1

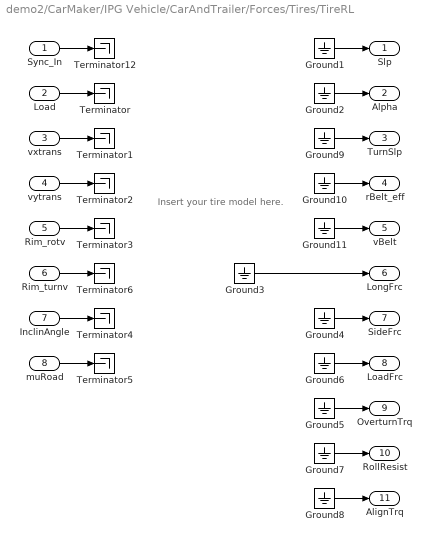
== system demo2/CarMaker/IPG Vehicle/CarAndTrailer/Forces/Tires/TireRL ==
  note: Insert your tire model here.
  Sync_In : Inport
  Load : Inport  Port=2
  vxtrans : Inport  Port=3
  vytrans : Inport  Port=4
  Rim_rotv : Inport  Port=5
  Rim_turnv : Inport  Port=6
  InclinAngle : Inport  Port=7
  muRoad : Inport  Port=8
  Ground{1..11} (11 alike) : Ground
  Terminator{,1..6,12} (8 alike) : Terminator
  Slp : Outport  VectorParamsAs1DForOutWhenUnconnected=off
  Alpha : Outport  Port=2  VectorParamsAs1DForOutWhenUnconnected=off
  TurnSlp : Outport  Port=3  VectorParamsAs1DForOutWhenUnconnected=off
  rBelt_eff : Outport  Port=4  VectorParamsAs1DForOutWhenUnconnected=off
  vBelt : Outport  Port=5  VectorParamsAs1DForOutWhenUnconnected=off
  LongFrc : Outport  Port=6  VectorParamsAs1DForOutWhenUnconnected=off
  SideFrc : Outport  Port=7  VectorParamsAs1DForOutWhenUnconnected=off
  LoadFrc : Outport  Port=8  VectorParamsAs1DForOutWhenUnconnected=off
  OverturnTrq : Outport  Port=9  VectorParamsAs1DForOutWhenUnconnected=off
  RollResist : Outport  Port=10  VectorParamsAs1DForOutWhenUnconnected=off
  AlignTrq : Outport  Port=11  VectorParamsAs1DForOutWhenUnconnected=off
  wires:
  Ground11/1 -> vBelt/1
  Ground10/1 -> rBelt_eff/1
  Ground9/1 -> TurnSlp/1
  Rim_turnv/1 -> Terminator6/1
  Sync_In/1 -> Terminator12/1
  Ground2/1 -> Alpha/1
  Ground4/1 -> SideFrc/1
  Ground5/1 -> OverturnTrq/1
  vxtrans/1 -> Terminator1/1
  vytrans/1 -> Terminator2/1
  Rim_rotv/1 -> Terminator3/1
  InclinAngle/1 -> Terminator4/1
  muRoad/1 -> Terminator5/1
  Load/1 -> Terminator/1
  Ground1/1 -> Slp/1
  Ground6/1 -> LoadFrc/1
  Ground7/1 -> RollResist/1
  Ground8/1 -> AlignTrq/1
  Ground3/1 -> LongFrc/1

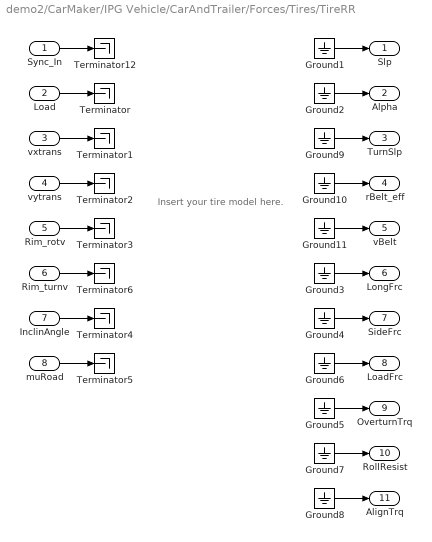
== system demo2/CarMaker/IPG Vehicle/CarAndTrailer/Forces/Tires/TireRR ==
  note: Insert your tire model here.
  Sync_In : Inport
  Load : Inport  Port=2
  vxtrans : Inport  Port=3
  vytrans : Inport  Port=4
  Rim_rotv : Inport  Port=5
  Rim_turnv : Inport  Port=6
  InclinAngle : Inport  Port=7
  muRoad : Inport  Port=8
  Ground{1..11} (11 alike) : Ground
  Terminator{,1..6,12} (8 alike) : Terminator
  Slp : Outport  VectorParamsAs1DForOutWhenUnconnected=off
  Alpha : Outport  Port=2  VectorParamsAs1DForOutWhenUnconnected=off
  TurnSlp : Outport  Port=3  VectorParamsAs1DForOutWhenUnconnected=off
  rBelt_eff : Outport  Port=4  VectorParamsAs1DForOutWhenUnconnected=off
  vBelt : Outport  Port=5  VectorParamsAs1DForOutWhenUnconnected=off
  LongFrc : Outport  Port=6  VectorParamsAs1DForOutWhenUnconnected=off
  SideFrc : Outport  Port=7  VectorParamsAs1DForOutWhenUnconnected=off
  LoadFrc : Outport  Port=8  VectorParamsAs1DForOutWhenUnconnected=off
  OverturnTrq : Outport  Port=9  VectorParamsAs1DForOutWhenUnconnected=off
  RollResist : Outport  Port=10  VectorParamsAs1DForOutWhenUnconnected=off
  AlignTrq : Outport  Port=11  VectorParamsAs1DForOutWhenUnconnected=off
  wires:
  Ground11/1 -> vBelt/1
  Ground10/1 -> rBelt_eff/1
  Ground9/1 -> TurnSlp/1
  Rim_turnv/1 -> Terminator6/1
  Sync_In/1 -> Terminator12/1
  Ground2/1 -> Alpha/1
  Ground3/1 -> LongFrc/1
  Ground4/1 -> SideFrc/1
  Ground5/1 -> OverturnTrq/1
  vxtrans/1 -> Terminator1/1
  vytrans/1 -> Terminator2/1
  Rim_rotv/1 -> Terminator3/1
  InclinAngle/1 -> Terminator4/1
  muRoad/1 -> Terminator5/1
  Load/1 -> Terminator/1
  Ground1/1 -> Slp/1
  Ground6/1 -> LoadFrc/1
  Ground7/1 -> RollResist/1
  Ground8/1 -> AlignTrq/1

== system demo2/CarMaker/VehicleControl/CreateBus VhclCtrl/MPC Controller/Adaptive MPC/Linearization ==
  operating state : Inport
  previous input : Inport  Port=2
  Terminator : Terminator
  Terminator1 : Terminator
  linearization : MATLAB Function  TreatAsAtomicUnit=on
  A : Outport
  B : Outport  Port=2
  C : Outport  Port=3
  wires:
  linearization/1(A) -> A/1
  linearization/2(B) -> B/1
  linearization/3(C) -> C/1
  linearization/4(D) -> Terminator1/1
  operating state/1 -> linearization/1(state)
  previous input/1 -> linearization/2(pre_input)
  linearization/5(DX) -> Terminator/1

== matlab function demo2/CarMaker/VehicleControl/CreateBus VhclCtrl/MATLAB Function3 ==
  data: u input; y output; v input
function y = fcn(u, v)

y = rem(u, pi/3);
y = tan(y);

y = y * v;

== matlab function demo2/CarMaker/VehicleControl/CreateBus VhclCtrl/MPC Controller/Adaptive MPC/Linearization/linearization ==
  data: state input; A output; B output; C output; D output; pre_input input; DX output; Cf parameter; Cr parameter; m parameter; Iz parameter; lf parameter; lr parameter; w parameter
function [A, B, C, D, DX] = fcn(state, pre_input, Cf, Cr, m, Iz, lf, lr, w)
% Start ========================================================================================
% [A,B,C,D] = CMmodel2_2(state,pre_input);
% ==============================================================================================
Vx = state(1);
Vy = state(2);
YawRate = state(3);

delta = pre_input(1);
%    Frxl = pre_input(2);
%    Frxr = pre_input(3);

dfdx_op = [

[                                               -(2*Cf*sin(delta)*(Vy + lf*YawRate))/(m*Vx^2),             YawRate + (2*Cf*sin(delta))/(m*Vx),                   Vy + (2*Cf*lf*sin(delta))/(m*Vx)]
[((2*Cr*(Vy - lr*YawRate))/Vx^2 + (2*Cf*cos(delta)*(Vy + lf*YawRate))/Vx^2)/m - YawRate,       -((2*Cr)/Vx + (2*Cf*cos(delta))/Vx)/m, ((2*Cr*lr)/Vx - (2*Cf*lf*cos(delta))/Vx)/m - Vx]
[  -((2*Cr*lr*(Vy - lr*YawRate))/Vx^2 - (2*Cf*lf*cos(delta)*(Vy + lf*YawRate))/Vx^2)/Iz, ((2*Cr*lr)/Vx - (2*Cf*lf*cos(delta))/Vx)/Iz,   -((2*Cf*cos(delta)*lf^2)/Vx + (2*Cr*lr^2)/Vx)/Iz]

];

dfdu_op = [

[      -(2*Cf*sin(delta) + 2*Cf*cos(delta)*(delta - (Vy + lf*YawRate)/Vx))/m,   1/m,  1/m]
[       (2*Cf*cos(delta) - 2*Cf*sin(delta)*(delta - (Vy + lf*YawRate)/Vx))/m,     0,    0]
[(2*Cf*lf*cos(delta) - 2*Cf*lf*sin(delta)*(delta - (Vy + lf*YawRate)/Vx))/Iz, -w/Iz, w/Iz]

];

A = dfdx_op;
B = dfdu_op;
C = eye(size(A));
D = zeros(size(B));

% End ==========================================================================================
% [A,B,C,D] = CMmodel2_2(state,pre_input);
% ==============================================================================================

DX = A*state + B*pre_input - state;
end

== matlab function demo2/CarMaker/VehicleControl/CreateBus VhclCtrl/MPC Controller/Adaptive MPC/MPC Main Function ==
  data: A input; B input; C input; state input; delState input; preInput input; U output [2..5]; ref input; Np parameter; Nc parameter; stateWeight parameter; controlWeight parameter; stateConstraints parameter; controlConstraints parameter; Ts parameter
function U = fcn(A,B,C, state, delState, preInput, ref, Np, Nc, stateWeight, controlWeight, stateConstraints, controlConstraints, Ts)
%% sixe
[stateSize, inputSize] = size(C);
augStateSize = stateSize * 2;
predStateSize = stateSize * Np;
predInputSize = inputSize * Nc;

%% model augmentation
augState = [delState; state];

% Start ========================================================================================
% [A,B,C,D] = augmentation_ext(A,B,C,D,Ts);
% ==============================================================================================
A = A*Ts+eye(stateSize);
B = B*Ts;

A = [A zeros(inputSize, stateSize);
    C*A eye(stateSize)];
B = [B; C*B];
C = [zeros(stateSize, inputSize) eye(stateSize)];
% End ==========================================================================================
% [A,B,C,D] = augmentation_ext(A,B,C,D,Ts);
% ==============================================================================================

%% weight matrices
stateWeight = reshape(stateWeight, 1, []);
stateWeight = repmat(stateWeight, 1, Np);

controlWeight = reshape(controlWeight, 1, []);
controlWeight = repmat(controlWeight, 1, Nc);

Q = diag(stateWeight);
R = diag(controlWeight);

%% Prediction Matrices and Vectors 
% reference vector
ref = repmat(ref,Np,1);

% Start ========================================================================================
% [F, Phi] = predMat(A, B, C, Np, Nc);
% ==============================================================================================
F = ones(predStateSize, augStateSize);
Phi = zeros(predStateSize, predInputSize);

for i = 1:1:Np
    F((i-1)*stateSize+1:i*stateSize, ...
        1:augStateSize) = C * A^i;
    for j = 1:1:Nc
        tmp = C * A^(i-1) * B;
        Phi((i+j-2)*stateSize+1:(i+j-1)*stateSize, ...
            (j-1)*inputSize+1:j*inputSize) = tmp;
    end
end

Phi = Phi(1:predStateSize,1:predInputSize);
% End ==========================================================================================
% [F, Phi] = predMat(A, B, C, Np, Nc);
% ==============================================================================================
H = Phi' * Q * Phi + R;
f = 2 * (ref - F * augState)' * Q * (-Phi);

if ~issymmetric(H)
    H = (H+H')/2;
end

%% constraints matrices
% Start ========================================================================================
% [a, b] = constraintMatrix(state, pre_input, Np, Nc, F, Phi, stateConstraints, controlConstraints);
% ==============================================================================================
% S1 = eye(input_size  * controlHorizon);
% S2 = tril(ones(size(S1)),-1) - tril(ones(size(S1)), -2);

C1 = eye(predInputSize);
C2 = tril(ones(size(C1)));

controlConstraints = reshape(controlConstraints, [], 4);
stateConstraints = reshape(stateConstraints, [], 4);

% a1 = []; b1 = [];

a2 = [Phi; -Phi];
b2 = [
    +repmat(stateConstraints(:,4), Np, 1) - F * augState;
    -repmat(stateConstraints(:,3), Np, 1) + F * augState
];

% delList = [];
% for i = 1:stateSize 
%     if stateConstraints(i,3) == stateConstraints(i,4)
%         tmp = (1:stateSize:predStateSize) + (i-1);
%         delList = [delList, tmp, tmp + predStateSize];
%     end
% end
% a2(delList, :) = [];
% b2(delList, :) = [];

a3 = [C1; -C1];
b3 = [
    +repmat(controlConstraints(:,2), Nc, 1);
    -repmat(controlConstraints(:,1), Nc, 1)
];

% delList = [];
% for i = 1:inputSize 
%     if controlConstraints(i,1) == controlConstraints(i,2)
%         tmp = (1:inputSize:predInputSize) + (i-1);
%         delList = [delList, tmp, tmp + predInputSize];
%     end
% end
% a3(delList, :) = [];
% b3(delList, :) = [];
 
a4 = [C2; -C2];
b4 = [
    -repmat(preInput, Nc, 1) + repmat(controlConstraints(:,4), Nc, 1);
    +repmat(preInput, Nc, 1) - repmat(controlConstraints(:,3), Nc, 1)
];

% delList = [];
% for i = 1:inputSize 
%     if controlConstraints(i,3) == controlConstraints(i,4)
%         tmp = (1:inputSize:predInputSize) + (i-1);
%         delList = [delList, tmp, tmp + predInputSize];
%     end
% end
% a4(delList, :) = [];
% b4(delList, :) = [];

a = [a2;a3;a4];
b = [b2;b3;b4];

% End ==========================================================================================
% [a, b] = constraintMatrix(state, pre_input, Np, Nc, F, Phi, stateConstraints, controlConstraints);
% ==============================================================================================

%% quadratic programming
options = optimoptions( ...
    'quadprog', ...
    'Algorithm','active-set', ...
    'Display','none' ...
    );

U = quadprog(H,f,a,b,[],[],[],[], preInput, options);
